simulink model "baro2altRen"  (Simulink 6.6)
settings: Solver=ode3  StartTime=0.0  StopTime=700  FixedStep=0.01  RelTol=1e-3
undefined symbols (not defined in the file or in its folder): AirDia
libraries: simulink x2, aerolibconvert2 x1
settings Model: Creator=Administrator  LastModifiedBy=Administrator

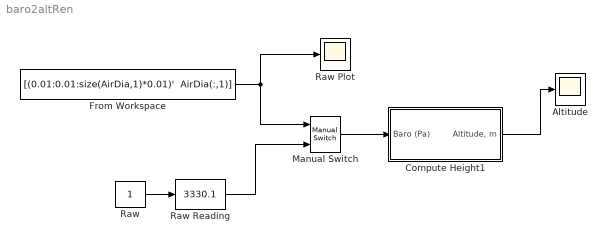
== system baro2altRen ==
  Altitude : Scope
      settings: TimeRange=700  YMin=117.0523317906728  YMax=134.5845496618013
  Compute Height1 : Subsystem  mask{basePressure=AirDia(1,1), baseTemp=288.215, LapseRate=-0.00198122, baseHeight=235}
      mask prompts: basePressure "Base Station Pressure (Pa)"; baseTemp "Base Station Temperature (K)"; LapseRate "Lapse Rate (C/ft)"; baseHeight "Base Station Known Height (m)"
      mask help:
      | Produces Altitude in meters from Raw Baro Altimeter. Altitude is valid from MSL to 6000 ft.
      |
      | The method implemented here was developed by Ren Curry
  From Workspace : FromWorkspace  VariableName="[(0.01:0.01:size(AirDia,1)*0.01)'  AirDia(:,1)]"  SampleTime=0.01
  Manual Switch : simulink/Signal Routing/Manual Switch  SystemSampleTime=-1  sw=1  action=0  varsize=off
  Raw : Constant
  Raw Plot : Scope
      settings: TimeRange=700  YMin=3258.205050999286  YMax=3359.639053031729
  Raw Reading : simulink/Math Operations/Slider Gain  SystemSampleTime=-1  low=0  gain=3330.1  high=4096
  wires:
  From Workspace/1 -> Raw Plot/1, Manual Switch/1
  Compute Height1/1("Altitude, m") -> Altitude/1
  Raw/1 -> Raw Reading/1
  Manual Switch/1 -> Compute Height1/1(Baro (Pa))
  Raw Reading/1 -> Manual Switch/2

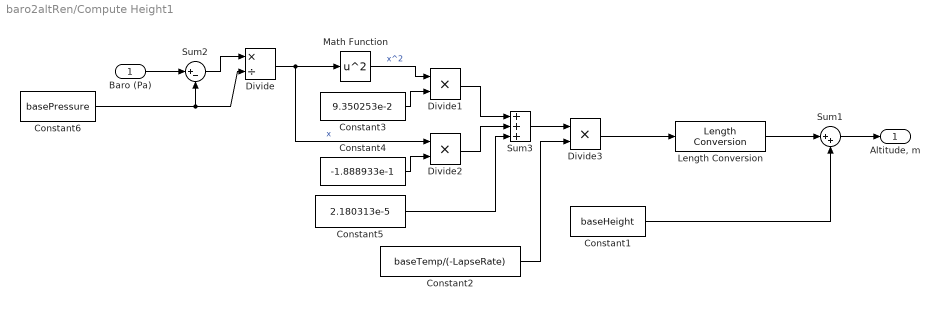
== system baro2altRen/Compute Height1 ==
  Baro (Pa) : Inport
  Constant1 : Constant  Value=baseHeight
  Constant2 : Constant  Value=baseTemp/(-LapseRate)
  Constant3 : Constant  Value=9.350253e-2
  Constant4 : Constant  Value=-1.888933e-1
  Constant5 : Constant  Value=2.180313e-5
  Constant6 : Constant  Value=basePressure
  Divide : Product  Inputs=*/  OutScaling=2^-10
  Divide1 : Product  OutScaling=2^-10
  Divide2 : Product  OutScaling=2^-10
  Divide3 : Product  OutScaling=2^-10
  Length Conversion : aerolibconvert2/Length Conversion  SystemSampleTime=-1  IU=ft  OU=m
  Math Function : Math  Operator=square  SaturateOnIntegerOverflow=on
  Sum1 : Sum  Inputs=|++
  Sum2 : Sum  Inputs=|+-
  Sum3 : Sum  Inputs=3
  "Altitude, m" : Outport
  wires:
  Length Conversion/1 -> Sum1/1
  Sum2/1 -> Divide/1
  Sum1/1 -> "Altitude, m"/1
  Divide3/1 -> Length Conversion/1
  Constant2/1 -> Divide3/2
  Sum3/1 -> Divide3/1
  Constant5/1 -> Sum3/3
  Divide2/1 -> Sum3/2
  Divide1/1 -> Sum3/1
  Constant4/1 -> Divide2/2
  Constant3/1 -> Divide1/2
  Math Function/1 -> Divide1/1  "x^2"
  Divide/1 -> Divide2/1, Math Function/1  "x"
  Constant6/1 -> Divide/2, Sum2/2
  Constant1/1 -> Sum1/2
  Baro (Pa)/1 -> Sum2/1
